simulink model "rest"  (R2020b)
settings: Solver=VariableStepAuto  StartTime=0.0  StopTime=10.0  RelTol=1e-3
undefined symbols (not defined in the file): B, Beta, kc, ke, ki, kp, M, w0, wu
settings Model: Creator=Laura  LastModifiedBy=Laura

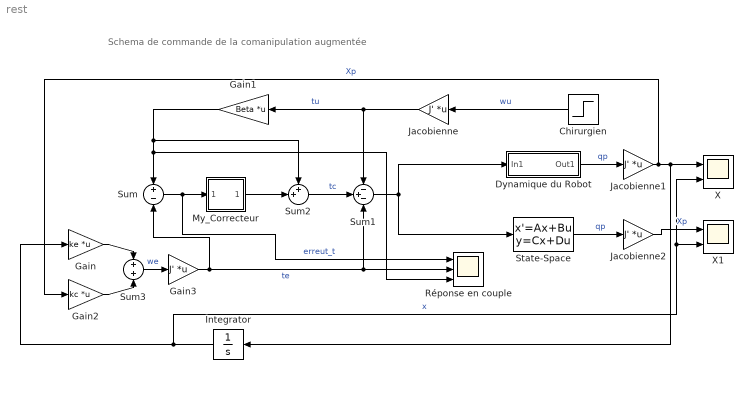
== system rest ==
  note: Schema de commande de la comanipulation augmentée
  Chirurgien : Step  Before=w0  After=wu  SampleTime=0  VectorParams1D=off
  Dynamique du Robot : Subsystem
      mask Display: disp('(Ms + B)^-1')
  Gain : Gain  Gain=ke  Multiplication=Matrix(K*u)
  Gain1 : Gain  Gain=Beta  Multiplication=Matrix(K*u)
  Gain2 : Gain  Gain=kc  Multiplication=Matrix(K*u)
  Gain3 : Gain  Gain=J'  Multiplication=Matrix(K*u)
  Integrator : Integrator
  Jacobienne : Gain  Gain=J'  Multiplication=Matrix(K*u)
  Jacobienne1 : Gain  Gain=J'  Multiplication=Matrix(K*u)
  Jacobienne2 : Gain  Gain=J'  Multiplication=Matrix(K*u)
  My_Correcteur : Subsystem
      mask Display: disp('PI')
  Réponse en couple : Scope  NumInputPorts=3
  State-Space : StateSpace  A=-M^-1*B  B=M^-1  C=eye(2)  D=zeros(2,2)  InitialCondition=0
  Sum : Sum  Inputs=+|-
  Sum1 : Sum  Inputs=-+-
  Sum2 : Sum  Inputs=++|
  Sum3 : Sum  Inputs=+|+
  X : Scope  NumInputPorts=2
  X1 : Scope  NumInputPorts=2
  wires:
  Gain3/1 -> Sum/2, Réponse en couple/2, Sum1/3  "te"
  Sum3/1 -> Gain3/1  "we"
  Sum1/1 -> Dynamique du Robot/1(In1), State-Space/1
  Dynamique du Robot/1(Out1) -> Jacobienne1/1  "qp"
  Chirurgien/1 -> Jacobienne/1  "wu"
  Jacobienne/1 -> Gain1/1, Sum1/1  "tu"
  Gain1/1 -> Sum2/1, Réponse en couple/3, Sum/1
  Sum2/1 -> Sum1/2  "tc"
  Jacobienne1/1 -> Integrator/1, X/1, Gain2/1  "Xp"
  Sum/1 -> My_Correcteur/1(erreut_t), Réponse en couple/1  "erreut_t"
  My_Correcteur/1(Out1) -> Sum2/2
  Jacobienne2/1 -> X1/1  "Xp"
  State-Space/1 -> Jacobienne2/1  "qp"
  Gain2/1 -> Sum3/2
  Gain/1 -> Sum3/1
  Integrator/1 -> X1/2, X/2, Gain/1  "x"

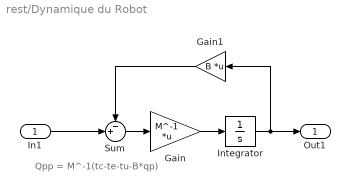
== system rest/Dynamique du Robot ==
  note: Qpp = M^-1(tc-te-tu-B*qp)
  In1 : Inport
  Gain : Gain  Gain=M^-1  Multiplication=Matrix(K*u)
  Gain1 : Gain  Gain=B  Multiplication=Matrix(K*u)
  Integrator : Integrator
  Sum : Sum  Inputs=-+|
  Out1 : Outport
  wires:
  Gain/1 -> Integrator/1
  Sum/1 -> Gain/1
  Gain1/1 -> Sum/1
  Integrator/1 -> Gain1/1, Out1/1
  In1/1 -> Sum/2

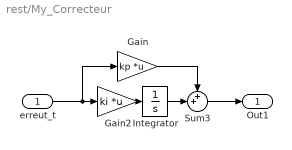
== system rest/My_Correcteur ==
  erreut_t : Inport
  Gain : Gain  Gain=kp  Multiplication=Matrix(K*u)
  Gain2 : Gain  Gain=ki  Multiplication=Matrix(K*u)
  Integrator : Integrator  InitialCondition=w0
  Sum3 : Sum  Inputs=++|
  Out1 : Outport
  wires:
  Sum3/1 -> Out1/1
  Gain/1 -> Sum3/1
  Gain2/1 -> Integrator/1
  Integrator/1 -> Sum3/2
  erreut_t/1 -> Gain/1, Gain2/1
